simulink model "untitled33333"  (R2017b)
settings: Solver=FixedStepAuto  StartTime=0.0  StopTime=2  FixedStep=0.002  RelTol=1e-3
libraries: simulink x9
settings Model: Creator=Admin  LastModifiedBy=Admin

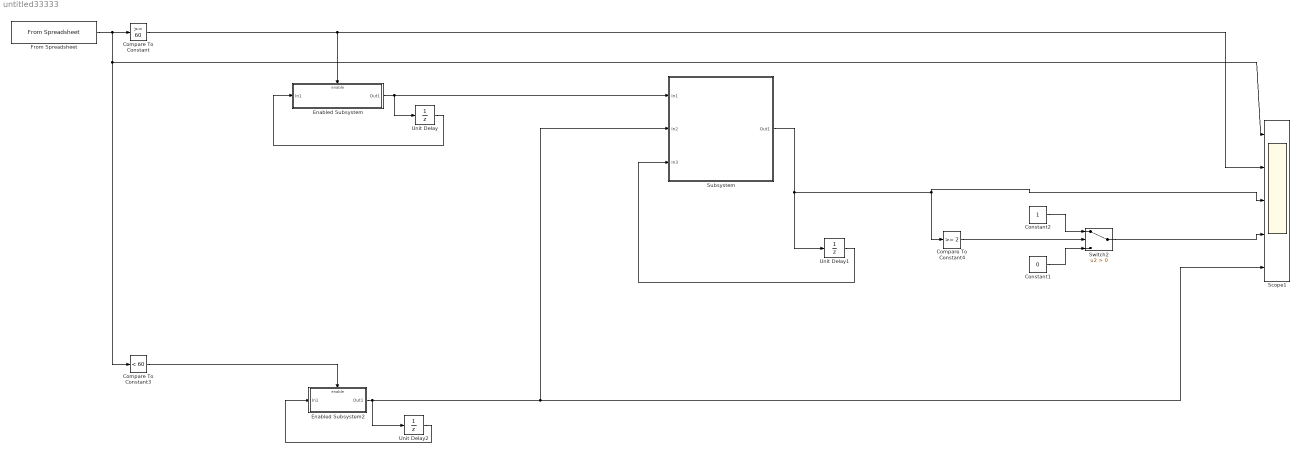
== system untitled33333 ==
  Compare To Constant : simulink/Logic and Bit Operations/Compare To Constant  relop=>=  const=60  OutDataTypeStr=boolean
  Compare To Constant3 : simulink/Logic and Bit Operations/Compare To Constant  relop=<  const=60  OutDataTypeStr=boolean
  Compare To Constant4 : simulink/Logic and Bit Operations/Compare To Constant  relop=>=  const=2  OutDataTypeStr=boolean
  Constant1 : Constant  Value=0
  Constant2 : Constant
  Enabled Subsystem : Subsystem  TreatAsAtomicUnit=on
  Enabled Subsystem2 : Subsystem  TreatAsAtomicUnit=on
  From Spreadsheet : FromSpreadsheet  FileName=dulieu.xlsx
  Scope1 : Scope  NumInputPorts=5
  Subsystem : Subsystem
  Switch2 : Switch  Criteria=u2 > Threshold
  Unit Delay : UnitDelay  SampleTime=-1
  Unit Delay1 : UnitDelay  SampleTime=-1
  Unit Delay2 : UnitDelay  SampleTime=-1
  wires:
  Compare To Constant/1 -> Enabled Subsystem/Enable, Scope1/2
  From Spreadsheet/1 -> Compare To Constant3/1, Scope1/1, Compare To Constant/1
  Unit Delay/1 -> Enabled Subsystem/1(In1)
  Compare To Constant3/1 -> Enabled Subsystem2/Enable
  Compare To Constant4/1 -> Switch2/2
  Constant2/1 -> Switch2/1
  Constant1/1 -> Switch2/3
  Switch2/1 -> Scope1/4
  Enabled Subsystem2/1(Out1) -> Subsystem/2(In2), Scope1/5, Unit Delay2/1
  Unit Delay2/1 -> Enabled Subsystem2/1(In1)
  Subsystem/1(Out1) -> Unit Delay1/1, Compare To Constant4/1, Scope1/3
  Enabled Subsystem/1(Out1) -> Unit Delay/1, Subsystem/1(In1)
  Unit Delay1/1 -> Subsystem/3(In3)

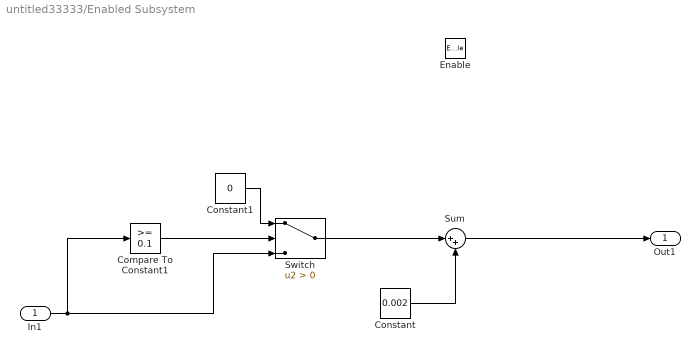
== system untitled33333/Enabled Subsystem ==
  In1 : Inport
  Enable : EnablePort  StatesWhenEnabling=reset
  Compare To Constant1 : simulink/Logic and Bit Operations/Compare To Constant  relop=>=  const=0.1  OutDataTypeStr=boolean
  Constant : Constant  Value=0.002
  Constant1 : Constant  Value=0
  Sum : Sum  Inputs=|++
  Switch : Switch  Criteria=u2 > Threshold
  Out1 : Outport  OutputWhenDisabled=reset  InitialOutput=0
  wires:
  Constant/1 -> Sum/2
  Sum/1 -> Out1/1
  In1/1 -> Compare To Constant1/1, Switch/3
  Constant1/1 -> Switch/1
  Switch/1 -> Sum/1
  Compare To Constant1/1 -> Switch/2

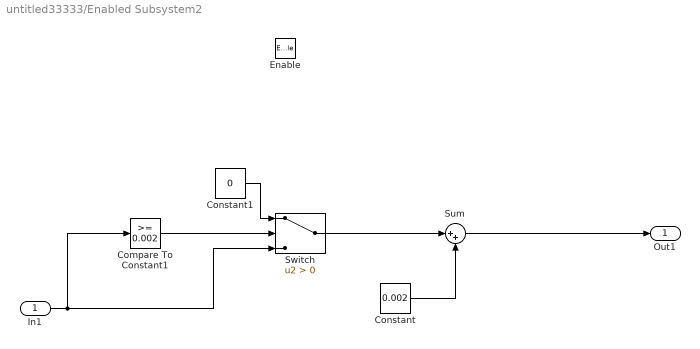
== system untitled33333/Enabled Subsystem2 ==
  In1 : Inport
  Enable : EnablePort
  Compare To Constant1 : simulink/Logic and Bit Operations/Compare To Constant  relop=>=  const=0.002  OutDataTypeStr=boolean
  Constant : Constant  Value=0.002
  Constant1 : Constant  Value=0
  Sum : Sum  Inputs=|++
  Switch : Switch  Criteria=u2 > Threshold
  Out1 : Outport  OutputWhenDisabled=reset  InitialOutput=0
  wires:
  Constant1/1 -> Switch/1
  Compare To Constant1/1 -> Switch/2
  Sum/1 -> Out1/1
  In1/1 -> Compare To Constant1/1, Switch/3
  Constant/1 -> Sum/2
  Switch/1 -> Sum/1

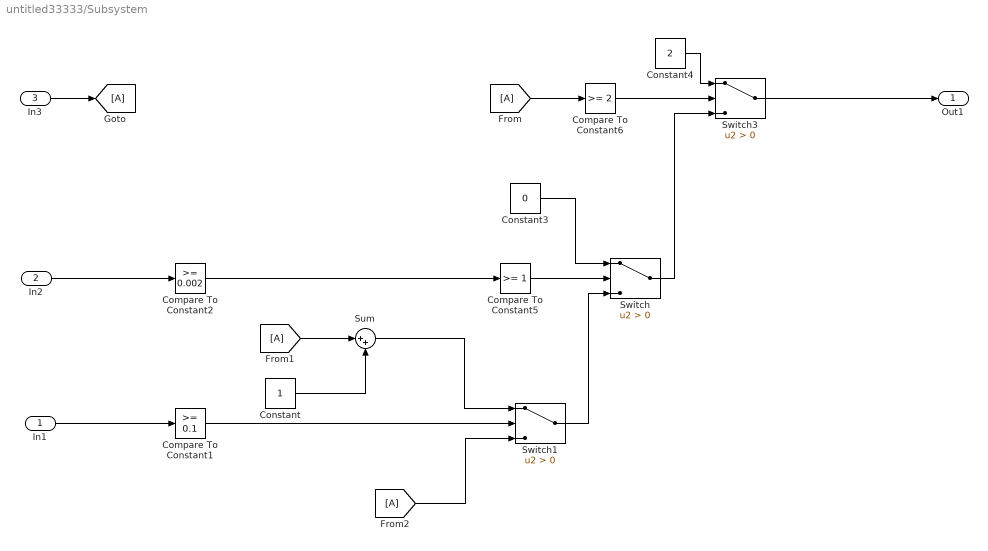
== system untitled33333/Subsystem ==
  In1 : Inport
  In2 : Inport  Port=2
  In3 : Inport  Port=3
  Compare To Constant1 : simulink/Logic and Bit Operations/Compare To Constant  relop=>=  const=0.1  OutDataTypeStr=boolean
  Compare To Constant2 : simulink/Logic and Bit Operations/Compare To Constant  relop=>=  const=0.002  OutDataTypeStr=boolean
  Compare To Constant5 : simulink/Logic and Bit Operations/Compare To Constant  relop=>=  const=1  OutDataTypeStr=boolean
  Compare To Constant6 : simulink/Logic and Bit Operations/Compare To Constant  relop=>=  const=2  OutDataTypeStr=boolean
  Constant : Constant
  Constant3 : Constant  Value=0
  Constant4 : Constant  Value=2
  Sum : Sum  Inputs=|++
  Switch : Switch  Criteria=u2 > Threshold
  Switch1 : Switch  Criteria=u2 > Threshold
  Switch3 : Switch  Criteria=u2 > Threshold
  Out1 : Outport
  wires:
  In2/1 -> Compare To Constant2/1
  Switch3/1 -> Out1/1
  Switch1/1 -> Switch/3
  Constant4/1 -> Switch3/1
  Compare To Constant5/1 -> Switch/2
  Constant3/1 -> Switch/1
  Constant/1 -> Sum/2
  Switch/1 -> Switch3/3
  Compare To Constant6/1 -> Switch3/2
  In1/1 -> Compare To Constant1/1
  Sum/1 -> Switch1/1
  Compare To Constant2/1 -> Compare To Constant5/1
  Compare To Constant1/1 -> Switch1/2
  In3/1 -> [A]
  [A] -> Compare To Constant6/1
  [A] -> Sum/1
  [A] -> Switch1/3
